simulink model "squaring"  (R2013a)
settings: Solver=VariableStepDiscrete  StartTime=0.0  StopTime=20  RelTol=1e-3
PreLoadFcn:
  | Fs = 1000;
  | Fd = 10;
StopFcn:
  | figure(1)
  | hold off
  | plot(Vss_nom,'b');
  | hold on
  | plot(Vss,'r');
  | legend('Centre SS', 'Adj. SS',0);
  | 
  | doFFTplot(Fs, [Vmod(round(length(Vmod)*0.5):end), Vfc(round(length(Vfc)*0.5):end), Vref(round(length(Vref)*0.5):end)], ['Input  '; 'Synth  '; 'Carrier'], 1, 2, 'hann');
  | doFFTplot(Fs, [Squared(2:end), Squared_Filt(2:end)], ['Squared'; 'SquareF'], 1, 3, 'hann');
  | 
  | figure(4)
  | hold off
  | plot(Vref,'b-o');
  | hold on
  | plot(Vfc,'r-o');
  | plot(zeros(1,length(Vref)),'k--');
  | axis([0 length(Vref) -(max(abs(Vref))*1.1) (max(abs(Vref))*1.1)]);
  | legend('Input Carrier','Output Sine',1)
  | 
  | figure(5)
  | hold off
  | plot(Vmod,'k-o');
  | hold on
  | plot(Vfc,'r-o');
  | plot(zeros(1,length(Vmod)),'k--');
  | axis([0 length(Vmod) -(max(abs(Vmod))*1.1) (max(abs(Vmod))*1.1)]);
  | legend('Modulated Input','Output Sine',1)
undefined symbols (not defined in the file): xlfda_numerator, xlipgetpartsetting
libraries: xbsIndex_r4 x26
settings Model: Creator=lcrockett  LastModifiedBy=hebin
settings DataIOCC: SignalLoggingSaveFormat=ModelDataLogs
settings OptimizationCC: ExpressionDepthLimit=2147483647  InitFltsAndDblsToZero=on
settings DebuggingCC: SaveWithParameterizedLinksMsg=none  FcnCallInpInsideContextMsg=UseLocalSettings  StrictBusMsg=Warning
settings GRTTargetCC: TargetFcnLib=ansi_tfl_tmw.mat  CombineOutputUpdateFcns=off  GRTInterface=on

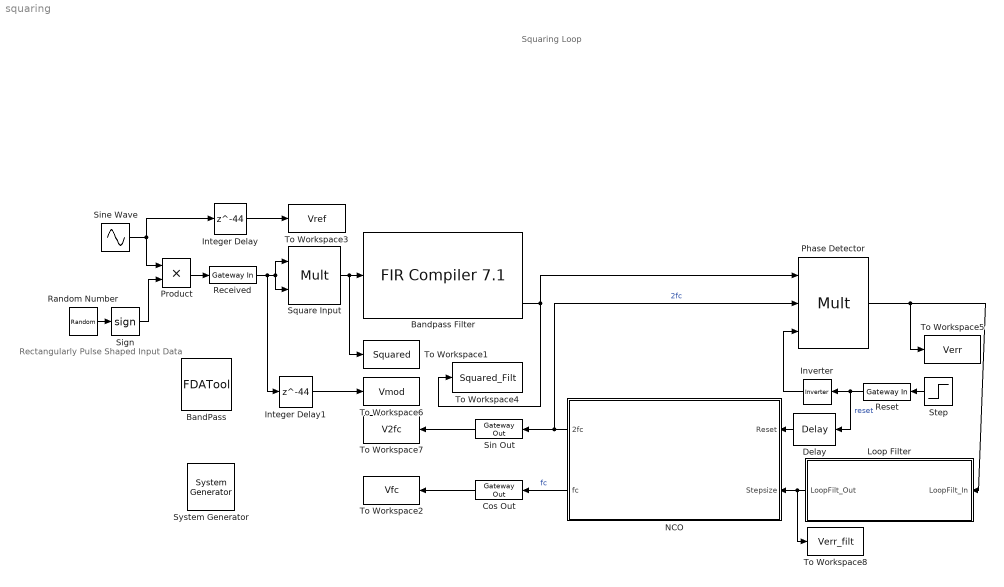
== system squaring ==
  note: Squaring Loop
  note: Rectangularly Pulse
      | Shaped Input Data
  " System Generator" : xbsIndex_r4/ System Generator  Tag=genX  xilinxfamily=kintex7  part=xc7k325t  speed=-3  package=fbg676  synthesis_tool=Vivado  clock_wrapper=Clock Enables  directory=./netlist  proj_type=Vivado  Synth_file=Vivado Synthesis Defaults  Impl_file=Vivado Implementation Defaults  testbench=off  simulink_period=1/Fs  sysclk_period=10  dcm_input_clock_period=10  incr_netlist=off  trim_vbits=Everywhere in SubSystem  dbl_ovrd=According to Block Masks  core_generation=According to Block Masks  run_coregen=off  deprecated_control=off  eval_field=0  block_type=sysgen
  BandPass : xbsIndex_r4/FDATool  block_type=fdatool
      settings: infoedit=FDATool
  "Bandpass Filter " : xbsIndex_r4/FIR Compiler 7.1   coefficientvector=xlfda_numerator('BandPass')  coefficient_sets=1  coefficient_reload=off  filter_type=Single_Rate  rate_change_type=Integer  interpolation_rate=1  decimation_rate=1  zero_pack_factor=1  channel_sequence=Basic  number_channels=1  pattern_list='P4-0,P4-1,P4-2,P4-3,P4-4'  number_paths=1  ratespecification=Hardware_Oversampling_Rate  sampleperiod=1  hardwareoversamplingrate=1  coefficient_sign=Signed  quantization=Quantize_Only  coefficient_width=16  bestprecision=on  coefficient_fractional_bits=14  coefficient_structure=Inferred  output_rounding_mode=Full_Precision  output_width=24  filter_architecture=Systolic_Multiply_Accumulate  optimization_goal=Area  optimization_list='None'  data_buffer_type=Automatic  coefficient_buffer_type=Automatic  input_buffer_type=Automatic  output_buffer_type=Automatic  preference_for_other_storage=Automatic  multi_column_support=Automatic  columnconfig='1'  inter_column_pipe_length=4  data_has_tlast=Not_Required  m_data_has_tready=off  s_data_has_fifo=off  s_data_has_tuser=Not_Required  m_data_has_tuser=Not_Required  s_config_sync_mode=On_Vector  s_config_method=Single  num_reload_slots=1  has_aclken=off  has_aresetn=off  infoeditControl=ARESETn must be asserted for a minimum of 2 cycles  trim_axipin_name=on  passband_min=0.0  passband_max=0.5  stopband_min=0.5  stopband_max=1.0  filter_selection=1  gui_behaviour=Sysgen_GUI  data_sign=Signed  data_width=16  data_fractional_bits=0  data_tuser_width=1  wrapper_available=true  ip_wrap_arbitrary_binary_point=true  ip_name=FIR Compiler  ip_version=7.1  dsptool_ready=true  ipcore_usecache=true  ipcore_useipmodelcache=true  ipcore_xco_need_fpga_part=true  port_translation_map={ 'aclken' => 'en', 'aresetn' => 'rst' }  run_core_at_system_period=true  ipcore_fpga_part=xlipgetpartsetting(gcb, {'kintex7', 'xc7k325t', '-3', 'fbg676'})  block_type=fir_compiler_v7_1
      settings: infoedit=Maximum Possible : Maximizes oversampling rate. Abstracted input handshake (no s_data_tvalid) and automatic rate propagation.<br>Hardware Oversampling Rate : Specifies oversampling rate relative to the input sample period. Abstracted input handshake (no s_data_tvalid) and automatic rate propagation.<br>Sample Period : Specifies absolute oversampling rate. No input handshake abstraction (exposes s_data_tvalid) and no rate propagation.
  Cos Out : xbsIndex_r4/Gateway Out  inherit_from_input=off  hdl_port=on  rows=1  columns=1  UseAsDAC=off  DACChannel='1'  interface=None  automatic_assignment=on  address_offset=hex2dec('00')  intf_description=''  timing_constraint=None  locs_specified=off  LOCs={}  io_standard={}  block_type=gatewayout
      settings: infoedit="Gateway out block.  Converts Xilinx fixed point inputs into ouputs of type Simulink integer, double, or fixed point.<P><P>Hardware notes:  In hardware these blocks become top level output ports or are discarded, depending on how they are configured."  block_version=9.2.01
  Delay : xbsIndex_r4/Delay  rst=off  infoeditControl=Selection of Reset will increase slice count due to use of real FFs and instead of SRLs  en=off  latency=1  reg_retiming=off  dbl_ovrd=off  block_type=delay
      settings: block_version=9.2.01
  Integer Delay : Delay  DelayLength=44  InputProcessing=Inherited
  Integer Delay1 : Delay  DelayLength=44  InputProcessing=Inherited
  Inverter : xbsIndex_r4/Inverter  en=off  latency=0  dbl_ovrd=off  block_type=inv
      settings: block_version=9.2.01
  Loop Filter : Subsystem  mask(Loop Filter Parameters){alpha_n=3, beta_n=7, phase_det_word=32, acc_ibits=10}
      mask prompts: alpha_n "Alpha (bits to shift right by)"; beta_n "Beta (bits to shift right by)"; phase_det_word "Input wordlength"; acc_ibits "Accumulator integer bits"
      mask help:
      | The loop filter contains two paths: a proportional path and an integral path. These have coefficients Alpha, and [Alpha x Beta], respectively.
      |
      | The wordlengths at the outputs of the shifts are extended by the degrees of the shifts. This also defines the number of fractional bits required in the accumulator of the integrator. The number of whole bits should be sufficient to prevent overflow.
      mask init:
      | alpha_shift_wl = phase_det_word + alpha_n;
      | beta_shift_wl = phase_det_word + beta_n;
  NCO : Subsystem  mask(Numerically Controlled Oscillator){N=1024, LUT_w=16, F_res=0.00001, F_nom=100, F_s=Fs}
      mask prompts: N "Lookup Table size, N (where N = 2^n)"; LUT_w "Lookup Table output wordlength"; F_res "Desired Frequency Resolution (Hz)"; F_nom "Desired Nominal frequency (Hz)"; F_s "Sampling frequency (Hz)"
      mask help: When specifying the resolution, ensure that the required number of fractional bits are available on the input data path (which provides the step size). Otherwise, the level of frequency resolution stated on the NCO block will not be realised.
      mask init:
      | delta_mu_des = (F_res * N) / F_s;
      | fract_bits = ceil(abs((log(delta_mu_des) / log(2))));
      | whole_bits = round(log(N)/log(2));
      | mu_nom = (F_nom * N) / F_s;
      | F_res_act = F_s / ((2^fract_bits) * N);
      mask Display: fprintf(['Actual Frequency Resolution = ', num2str(F_res_act), 'Hz\n Whole Bits = ', num2str(whole_bits), '\n Fractional Bits = ', num2str(fract_bits)],'texmode','on');
  Phase Detector : xbsIndex_r4/Mult  precision=Full  arith_type="Signed  (2's comp)"  n_bits=16  bin_pt=14  quantization=Truncate  overflow=Wrap  en=on  latency=1  use_behavioral_HDL=off  opt=Speed  use_embedded=on  optimum_pipeline=off  pipeline=on  dbl_ovrd=off  use_rpm=on  placement_style=Triangular  block_type=mult
      settings: infoedit=Hardware notes: To use the internal pipeline stage of the dedicated multiplier you must select 'Pipeline for maximum performance'.  block_version=9.2.01
  Product : Product  RndMeth=Zero
  Random Number : RandomNumber  Seed=90  SampleTime=1/Fd
  Received : xbsIndex_r4/Gateway In  gui_display_data_type=Fixed-point  arith_type="Signed  (2's comp)"  n_bits=16  bin_pt=14  preci_type=Single  exp_width=8  frac_width=24  quantization="Round  (unbiased: +/- Inf)"  overflow=Saturate  period=1/Fs  UseAsADC=off  ADCChannel='1'  interface=None  automatic_assignment=on  address_offset=hex2dec('00')  intf_description=''  timing_constraint=None  locs_specified=off  LOCs={}  inherit_from_input=off  hdl_port=on  dbl_ovrd=off  io_standard={}  block_type=gatewayin
      settings: infoedit="Gateway in block.  Converts inputs of type Simulink integer, double and fixed point to  Xilinx fixed point type.<P><P>Hardware notes:  In hardware these blocks become top level input ports."  block_version=9.2.01
  Reset : xbsIndex_r4/Gateway In  gui_display_data_type=Fixed-point  arith_type=Boolean  n_bits=16  bin_pt=14  preci_type=Single  exp_width=8  frac_width=24  quantization="Round  (unbiased: +/- Inf)"  overflow=Saturate  period=1/Fs  UseAsADC=off  ADCChannel='1'  interface=None  automatic_assignment=on  address_offset=hex2dec('00')  intf_description=''  timing_constraint=None  locs_specified=off  LOCs={}  inherit_from_input=off  hdl_port=on  dbl_ovrd=off  io_standard={}  block_type=gatewayin
      settings: infoedit="Gateway in block.  Converts inputs of type Simulink integer, double and fixed point to  Xilinx fixed point type.<P><P>Hardware notes:  In hardware these blocks become top level input ports."  block_version=9.2.01
  Sign : Signum
  Sin Out : xbsIndex_r4/Gateway Out  inherit_from_input=off  hdl_port=on  rows=1  columns=1  UseAsDAC=off  DACChannel='1'  interface=None  automatic_assignment=on  address_offset=hex2dec('00')  intf_description=''  timing_constraint=None  locs_specified=off  LOCs={}  io_standard={}  block_type=gatewayout
      settings: infoedit="Gateway out block.  Converts Xilinx fixed point inputs into ouputs of type Simulink integer, double, or fixed point.<P><P>Hardware notes:  In hardware these blocks become top level output ports or are discarded, depending on how they are configured."  block_version=9.2.01
  Sine Wave : Sin  Frequency=2*pi*96.77  SampleTime=1/Fs
  Square Input : xbsIndex_r4/Mult  precision=User Defined  arith_type="Signed  (2's comp)"  n_bits=16  bin_pt=14  quantization=Truncate  overflow=Wrap  en=off  latency=0  use_behavioral_HDL=off  opt=Speed  use_embedded=on  optimum_pipeline=off  pipeline=on  dbl_ovrd=off  use_rpm=on  placement_style=Triangular  block_type=mult
      settings: infoedit=Hardware notes: To use the internal pipeline stage of the dedicated multiplier you must select 'Pipeline for maximum performance'.  block_version=9.2.01
  Step : Step  Time=0.1  Before=1  After=0  SampleTime=2/Fs
  To Workspace1 : ToWorkspace  VariableName=Squared  SampleTime=-1
  To Workspace2 : ToWorkspace  VariableName=Vfc  SampleTime=-1
  To Workspace3 : ToWorkspace  VariableName=Vref  SampleTime=-1
  To Workspace4 : ToWorkspace  VariableName=Squared_Filt  SampleTime=-1
  To Workspace5 : ToWorkspace  VariableName=Verr  SampleTime=-1
  To Workspace6 : ToWorkspace  VariableName=Vmod  SampleTime=-1
  To Workspace7 : ToWorkspace  VariableName=V2fc  SampleTime=-1
  To Workspace8 : ToWorkspace  VariableName=Verr_filt  SampleTime=-1
  wires:
  NCO/2(fc) -> Cos Out/1  "fc"
  Received/1 -> Square Input/1, Square Input/2, Integer Delay1/1
  Square Input/1 -> "Bandpass Filter "/1, To Workspace1/1
  NCO/1(2fc) -> Sin Out/1, Phase Detector/2  "2fc"
  Cos Out/1 -> To Workspace2/1
  Product/1 -> Received/1
  Loop Filter/1(LoopFilt_Out) -> To Workspace8/1, NCO/2(Stepsize)
  Random Number/1 -> Sign/1
  Delay/1 -> NCO/1(Reset)
  Sine Wave/1 -> Product/1, Integer Delay/1
  Sign/1 -> Product/2
  Sin Out/1 -> To Workspace7/1
  Step/1 -> Reset/1
  Reset/1 -> Delay/1, Inverter/1  "reset"
  Phase Detector/1 -> Loop Filter/1(LoopFilt_In), To Workspace5/1
  Inverter/1 -> Phase Detector/3
  Integer Delay/1 -> To Workspace3/1
  Integer Delay1/1 -> To Workspace6/1
  "Bandpass Filter "/3 -> Phase Detector/1, To Workspace4/1

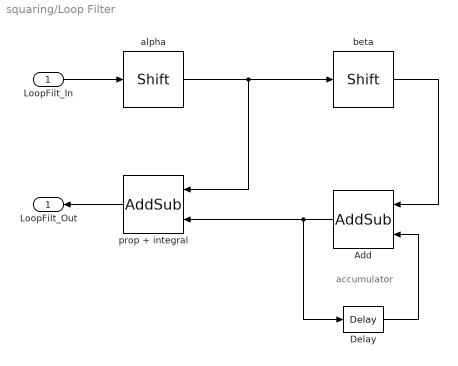
== system squaring/Loop Filter ==
  note: accumulator
  LoopFilt_In : Inport
  Add : xbsIndex_r4/AddSub  mode=Addition  use_carryin=off  use_carryout=off  en=off  latency=0  precision=User Defined  arith_type="Signed  (2's comp)"  n_bits=acc_ibits+beta_shift_wl-2  bin_pt=beta_shift_wl-2  quantization="Round  (unbiased: +/- Inf)"  overflow=Wrap  use_behavioral_HDL=off  hw_selection=Fabric  pipelined=off  use_rpm=on  dbl_ovrd=off  block_type=addsub
      settings: block_version=9.2.01
  Delay : xbsIndex_r4/Delay  rst=off  infoeditControl=Selection of Reset will increase slice count due to use of real FFs and instead of SRLs  en=off  latency=1  reg_retiming=off  dbl_ovrd=off  block_type=delay
      settings: block_version=9.2.01
  alpha : xbsIndex_r4/Shift  shift_dir=Right  shift_bits=alpha_n  en=off  latency=0  precision=User Defined  arith_type="Signed  (2's comp)"  n_bits=alpha_shift_wl  bin_pt=alpha_shift_wl-2  quantization=Truncate  overflow=Wrap  dbl_ovrd=off  block_type=shift
      settings: block_version=9.2.01
  beta : xbsIndex_r4/Shift  shift_dir=Right  shift_bits=beta_n  en=off  latency=0  precision=User Defined  arith_type="Signed  (2's comp)"  n_bits=beta_shift_wl  bin_pt=beta_shift_wl-2  quantization=Truncate  overflow=Wrap  dbl_ovrd=off  block_type=shift
      settings: block_version=9.2.01
  prop + integral : xbsIndex_r4/AddSub  mode=Addition  use_carryin=off  use_carryout=off  en=off  latency=0  precision=Full  arith_type="Signed  (2's comp)"  n_bits=20  bin_pt=14  quantization="Round  (unbiased: +/- Inf)"  overflow=Wrap  use_behavioral_HDL=off  hw_selection=Fabric  pipelined=off  use_rpm=on  dbl_ovrd=off  block_type=addsub
      settings: block_version=9.2.01
  LoopFilt_Out : Outport
  wires:
  Add/1 -> Delay/1, prop + integral/2
  Delay/1 -> Add/2
  LoopFilt_In/1 -> alpha/1
  prop + integral/1 -> LoopFilt_Out/1
  alpha/1 -> prop + integral/1, beta/1
  beta/1 -> Add/1

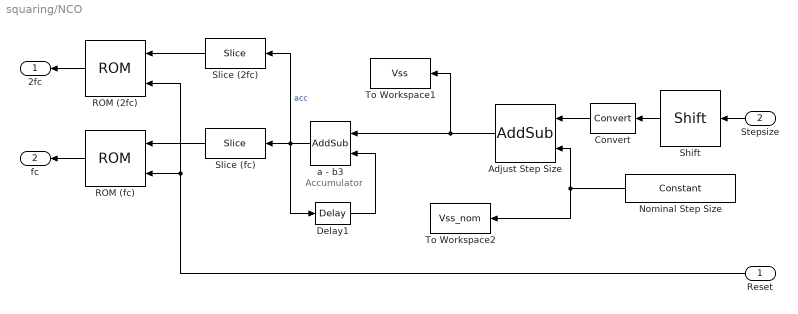
== system squaring/NCO ==
  note: Accumulator
  Reset : Inport
  Stepsize : Inport  Port=2
  Adjust Step Size : xbsIndex_r4/AddSub  mode=Addition  use_carryin=off  use_carryout=off  en=off  latency=0  precision=User Defined  arith_type=Unsigned  n_bits=whole_bits + fract_bits  bin_pt=fract_bits  quantization="Round  (unbiased: +/- Inf)"  overflow=Wrap  use_behavioral_HDL=off  hw_selection=Fabric  pipelined=off  use_rpm=on  dbl_ovrd=off  block_type=addsub
      settings: block_version=9.2.01
  Convert : xbsIndex_r4/Convert  gui_display_data_type=Fixed-point  arith_type="Signed  (2's comp)"  n_bits=whole_bits+fract_bits  bin_pt=fract_bits  float_type=Single  exp_bits=8  fraction_bits=24  quantization=Truncate  overflow=Wrap  en=off  latency=0  pipeline=off  dbl_ovrd=off  block_type=convert
      settings: block_version=9.2.01
  Delay1 : xbsIndex_r4/Delay  rst=off  infoeditControl=Selection of Reset will increase slice count due to use of real FFs and instead of SRLs  en=off  latency=1  reg_retiming=off  dbl_ovrd=off  block_type=delay
      settings: block_version=9.2.01
  Nominal Step Size : xbsIndex_r4/Constant  const=mu_nom  gui_display_data_type=Fixed-point  arith_type=Unsigned  n_bits=whole_bits + fract_bits  bin_pt=fract_bits  preci_type=Single  exp_width=8  frac_width=24  explicit_period=on  period=1/Fs  equ=P=C  opselect=C  inp2=PCIN>>17  opr=+  inp1=P  carry=CIN  dbl_ovrd=off  block_type=constant
      settings: block_version=9.2.01
  ROM (2fc) : xbsIndex_r4/ROM  depth=N  initVector=sin(pi*(0:(N-1))/(N/2))  distributed_mem=Block RAM  rst=on  init_reg=1  en=off  latency=1  gui_display_data_type=Fixed-point  arith_type="Signed  (2's comp)"  n_bits=LUT_w  bin_pt=LUT_w - 2  preci_type=Single  exp_width=8  frac_width=24  optimize=Area  use_rpm=on  dbl_ovrd=off  block_type=sprom
      settings: block_version=9.2.01
  ROM (fc) : xbsIndex_r4/ROM  depth=N  initVector=sin(pi*(0:(N-1))/(N/2))  distributed_mem=Block RAM  rst=on  init_reg=1  en=off  latency=1  gui_display_data_type=Fixed-point  arith_type="Signed  (2's comp)"  n_bits=LUT_w  bin_pt=LUT_w - 2  preci_type=Single  exp_width=8  frac_width=24  optimize=Area  use_rpm=on  dbl_ovrd=off  block_type=sprom
      settings: block_version=9.2.01
  Shift : xbsIndex_r4/Shift  shift_dir=Left  shift_bits=4  en=off  latency=0  precision=Full  arith_type="Signed  (2's comp)"  n_bits=16  bin_pt=14  quantization=Truncate  overflow=Wrap  dbl_ovrd=off  block_type=shift
      settings: block_version=9.2.01
  Slice (2fc) : xbsIndex_r4/Slice  nbits=whole_bits  boolean_output=off  mode=Upper Bit Location + Width  bit1=-1  base1=MSB of Input  bit0=0  base0=LSB of Input  dbl_ovrd=off  block_type=slice
      settings: infoedit="Extracts a given range of bits from each input sample and presents it at the output.  The output type is ordinarily unsigned with binary point at zero, but can be Boolean when the slice is one bit wide.<P><P>Hardware notes: In hardware this block costs nothing."  block_version=10.1
  Slice (fc) : xbsIndex_r4/Slice  nbits=whole_bits  boolean_output=off  mode=Upper Bit Location + Width  bit1=0  base1=MSB of Input  bit0=0  base0=LSB of Input  dbl_ovrd=off  block_type=slice
      settings: infoedit="Extracts a given range of bits from each input sample and presents it at the output.  The output type is ordinarily unsigned with binary point at zero, but can be Boolean when the slice is one bit wide.<P><P>Hardware notes: In hardware this block costs nothing."  block_version=10.1
  To Workspace1 : ToWorkspace  VariableName=Vss  SampleTime=-1
  To Workspace2 : ToWorkspace  VariableName=Vss_nom  SampleTime=-1
  a - b3 : xbsIndex_r4/AddSub  mode=Addition  use_carryin=off  use_carryout=off  en=off  latency=0  precision=User Defined  arith_type=Unsigned  n_bits=whole_bits + fract_bits  bin_pt=fract_bits  quantization=Truncate  overflow=Wrap  use_behavioral_HDL=off  hw_selection=Fabric  pipelined=off  use_rpm=on  dbl_ovrd=off  block_type=addsub
      settings: block_version=9.2.01
  2fc : Outport
  fc : Outport  Port=2
  wires:
  a - b3/1 -> Delay1/1, Slice (fc)/1, Slice (2fc)/1  "acc"
  Delay1/1 -> a - b3/2
  Slice (fc)/1 -> ROM (fc)/1
  ROM (fc)/1 -> fc/1
  Stepsize/1 -> Shift/1
  Reset/1 -> ROM (fc)/2, ROM (2fc)/2
  Adjust Step Size/1 -> a - b3/1, To Workspace1/1
  Nominal Step Size/1 -> Adjust Step Size/2, To Workspace2/1
  ROM (2fc)/1 -> 2fc/1
  Shift/1 -> Convert/1
  Convert/1 -> Adjust Step Size/1
  Slice (2fc)/1 -> ROM (2fc)/1
